simulink model "SPWM_19"  (R2019b)
settings: Solver=VariableStepAuto  StartTime=0.0  StopTime=0.1  RelTol=1e-3
libraries: powerlib x9, powerlib_meascontrol x1, simulink x1
settings Model: Creator=AASHYA  LastModifiedBy=swaga
settings DataIOCC: ReturnWorkspaceOutputs=off
settings SFSimCC: CustomCodeUndefinedFunction=UseInterfaceOnly

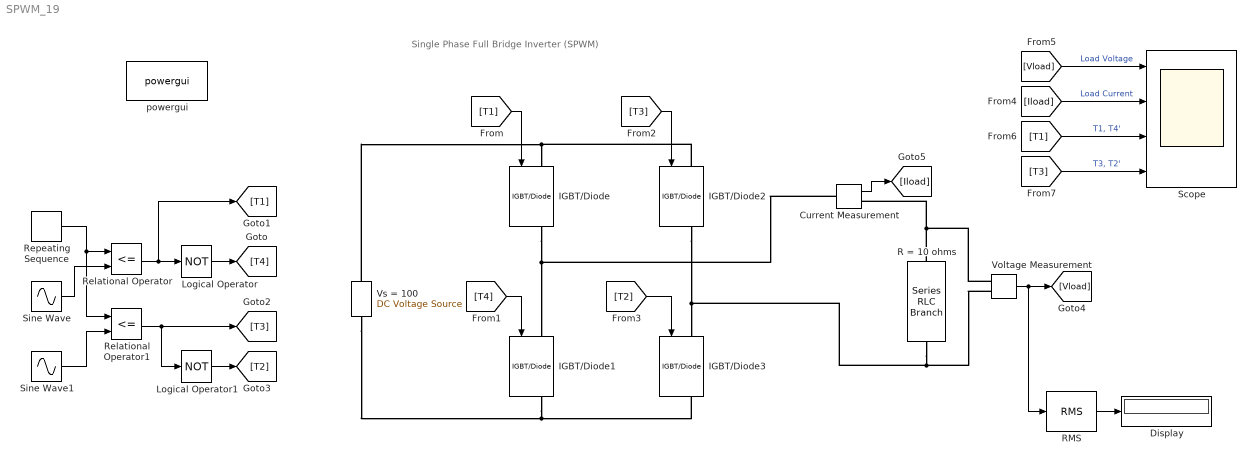
== system SPWM_19 ==
  note: Single Phase Full Bridge Inverter (SPWM)
  Current Measurement : powerlib/Measurements/Current Measurement  PhasorSimulation=off  OutputType=Complex  PSBequivalent=0
      settings: SourceProductName=Simscape Electrical
  Display : Display
  IGBT/Diode{,1..3} (4 alike) : powerlib/Power Electronics/IGBT//Diode  Ron=1e-3  Rs=1e5  Cs=inf  Measurements=on
      settings: SourceProductName=Simscape Electrical
  Logical Operator : Logic  Operator=NOT  AllPortsSameDT=off  OutDataTypeStr=boolean
  Logical Operator1 : Logic  Operator=NOT  AllPortsSameDT=off  OutDataTypeStr=boolean
  R = 10 ohms : powerlib/Elements/Series RLC Branch  LConnTagsString=__new0  RConnTagsString=__new0  BranchType=R  Resistance=10  Inductance=1e-3  SetiL0=off  InitialCurrent=0  Capacitance=1e-6  Setx0=off  InitialVoltage=0  Measurements=None
      settings: SourceProductName=Simscape Electrical
  RMS : powerlib_meascontrol/Measurements/RMS  TrueRMS=on  Freq=50  RMSInit=120  Ts=0
      settings: SourceProductName=Simscape Electrical
  Relational Operator : RelationalOperator  Operator=<=  OutDataTypeStr=boolean  RndMeth=Simplest
  Relational Operator1 : RelationalOperator  Operator=<=  OutDataTypeStr=boolean  RndMeth=Simplest
  Repeating Sequence : simulink/Sources/Repeating Sequence  rep_seq_t=[0 0.001]  rep_seq_y=[0 1]
  Scope : Scope  NumInputPorts=4
  Sine Wave : Sin  Amplitude=0.7  Frequency=2*pi*50  SampleTime=0
  Sine Wave1 : Sin  Amplitude=0.7  Frequency=2*pi*50  Phase=-pi  SampleTime=0
  Voltage Measurement : powerlib/Measurements/Voltage Measurement  PhasorSimulation=off  OutputType=Complex  PSBequivalent=0
      settings: SourceProductName=Simscape Electrical
  Vs = 100 : powerlib/Electrical Sources/DC Voltage Source  Amplitude=100  Measurements=None
      settings: SourceProductName=Simscape Electrical
  powergui : powerlib/powergui  Priority=1  SimulationMode=Discrete  SampleTime=5e-05  frequency=60  Iterations=50  frequencyindice=0  Pbase=100e6  ErrMax=1e-4  UnitsV=kV  UnitsW=MW  buscounter=0  FunctionMessages=off  echomessages=off  EnableUseOfTLC=off  CurrentSourceSwitches=off  DisableSnubberDevices=off  DisableRonSwitches=off  DisableVfSwitches=off  DisplayEquations=off  AutomaticDiscreteSolvers=off  SolverType=Tustin/Backward Euler (TBE)  Interpol=off  ExternalGateDelay=off  methode=off  Ts=100  x0status=blocks  SPID=on  SwTol=0  HookPort=off  NonlinearTolerance=1e-4  nMaxIteration=100  ContinueOnMaxIteration=off  RestoreLinks=warning  ResistiveCurrentMeasurement=off  Frange=[0:2:500]  Ylog=off  Xlog=on  ShowGrid=off  save=off  variable=ZData  structure=SquareWave  ZoomFFT=off  StartTime=0.0  cycles=1  DisplayStyle=1  fundamental=60  FreqAxis=off  MaxFrequency=1000  frequencyindicesteady=1  RmsSteady=1  display=off
      settings: SourceProductName=Simscape Electrical
  wires:
  RMS/1 -> Display/1
  Repeating Sequence/1 -> Relational Operator1/1, Relational Operator/1
  Sine Wave1/1 -> Relational Operator1/2
  Sine Wave/1 -> Relational Operator/2
  Relational Operator1/1 -> [T3], Logical Operator1/1
  Logical Operator/1 -> [T4]
  Relational Operator/1 -> [T1], Logical Operator/1
  Logical Operator1/1 -> [T2]
  Current Measurement/1 -> [Iload]
  Voltage Measurement/1 -> RMS/1, [Vload]
  [T1] -> IGBT/Diode/1
  [T4] -> IGBT/Diode1/1
  [T3] -> IGBT/Diode2/1
  [T2] -> IGBT/Diode3/1
  [Vload] -> Scope/1  "Load Voltage"
  [Iload] -> Scope/2  "Load Current"
  [T1] -> Scope/3  "T1, T4'"
  [T3] -> Scope/4  "T3, T2'"
  connections:
  IGBT/Diode/RConn1 -- Current Measurement/LConn1 -- IGBT/Diode1/LConn1
  IGBT/Diode2/RConn1 -- Voltage Measurement/LConn2 -- R = 10 ohms/RConn1 -- IGBT/Diode3/LConn1
  R = 10 ohms/LConn1 -- Voltage Measurement/LConn1 -- Current Measurement/RConn1
  IGBT/Diode2/LConn1 -- Vs = 100/RConn1 -- IGBT/Diode/LConn1
  IGBT/Diode1/RConn1 -- Vs = 100/LConn1 -- IGBT/Diode3/RConn1
